simulink model "speedgoat_test_SN5659_R2021b_IO612"  (R2021b)
settings: Solver=FixedStepDiscrete  StartTime=0.0  StopTime=20  RelTol=1e-3
PreLoadFcn:
  | Ts_IO107 = 0.001;
  | Ts_IO107 = 0.001;
  | Ts_IO133 = 0.001
  | 
  | Ts_IO204 = 0.001;
  | 
  | 
  | Ts_IO503 = 0.01;
  | 
  | ts_IO612 = 1e-3;
  | Ts_IO682 = 0.005;
  | Ts_IO941 = 0.01;
InitFcn:
  | Ts_IO107 = 0.001;
  | Ts_IO107 = 0.001;
  | Ts_IO133 = 0.001
  | 
  | Ts_IO204 = 0.001;
  | 
  | 
  | Ts_IO503 = 0.01;
  | 
  | ts_IO612 = 1e-3;
  | Ts_IO682 = 0.005;
  | Ts_IO941 = 0.01;
StopFcn:
  | if isfile(['sdi_view_',bdroot,'.mldatx'])
  |  Simulink.sdi.clearPreferences();
  |  Simulink.sdi.view();
  |  pause(3);
  |  Simulink.sdi.loadView(['sdi_view_',bdroot,]);
  | end
undefined symbols (not defined in the file): C
libraries: canmsglib x12, speedgoatlib_IO612 x9, simulink x1
settings Model: Creator=yannick.orgas  LastModifiedBy=ACH
settings SolverCC: ConcurrentTasks=on  AlgebraicLoopSolver=TrustRegion  PositivePriorityOrder=on
settings DataIOCC: LimitDataPoints=on  SaveFormat=StructureWithTime
settings OptimizationCC: BlockReduction=off  OptimizeBlockIOStorage=off
settings DebuggingCC: TasksWithSamePriorityMsg=none  UnconnectedInputMsg=none  UnconnectedOutputMsg=none  UnconnectedLineMsg=none  SFMachineParentedDataDiag=warning
settings HardwareCC: ProdBitPerLong=64  ProdLongLongMode=on  ProdHWDeviceType=Intel->x86-64 (Linux 64)
settings RTWCC: Description=Simulink Real-Time  SystemTargetFile=slrealtime.tlc  TemplateMakefile=slrealtime_default_tmf  Toolchain=Simulink Real-Time Toolchain  BuildConfiguration=Faster Runs  CodeExecutionProfiling=on  TargetLang=C++
settings SimulinkRealTimeTargetCC: UseGCCFastMath=on

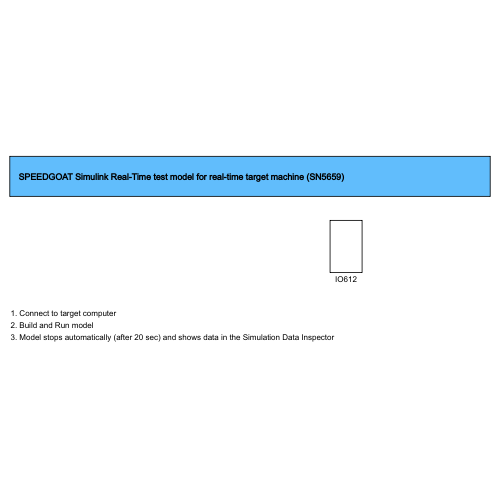
[thumbnail: Simulink's stored preview of the top-level diagram]
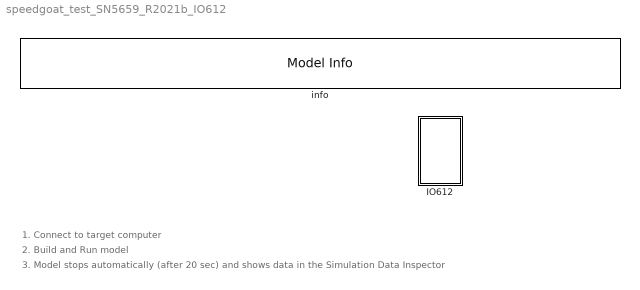
== system speedgoat_test_SN5659_R2021b_IO612 ==
  note: 1. Connect to target computer
  note: 2. Build and Run model
  note: 3. Model stops automatically (after 20 sec) and shows data in the Simulation Data Inspector
  IO612 : Subsystem
  info : simulink/Model-Wide Utilities/Model Info  Frame=on  DisplayStringWithTags=SPEEDGOAT Simulink Real-Time test model for real-time target machine (SN5659)  HorizontalTextAlignment=Left  LeftAlignmentValue=0.02

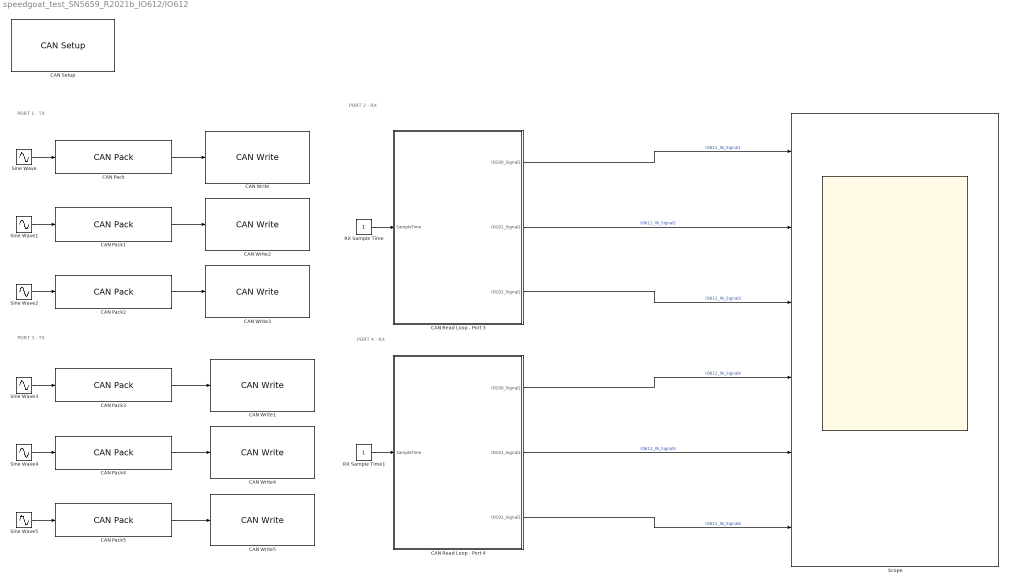
== system speedgoat_test_SN5659_R2021b_IO612/IO612 ==
  note: PORT 4 - RX
  note: PORT 1 - TX
  note: PORT 3 - TX
  note: PORT 2 - RX
  CAN Pack : canmsglib/CAN Pack  MsgList=(none)  MsgName=CAN Msg  MsgIDType=Standard (11-bit identifier)  MsgIdentifier=100  MsgLength=8  Remote=off  ApplyMinMax=off  BusOutput=off  SignalInfo={'Signal1','0','64','LE','double','Standard','0','1','0','-Inf','Inf'}
      settings: SourceProductBaseCode=ME,XP,VN  DataFormat=manually specified signals
  CAN Pack1 : canmsglib/CAN Pack  MsgList=(none)  MsgName=CAN Msg  MsgIDType=Standard (11-bit identifier)  MsgIdentifier=101  MsgLength=8  Remote=off  ApplyMinMax=off  BusOutput=off  SignalInfo={'Signal1','0','64','LE','double','Standard','0','1','0','-Inf','Inf'}
      settings: SourceProductBaseCode=ME,XP,VN  DataFormat=manually specified signals
  CAN Pack2 : canmsglib/CAN Pack  MsgList=(none)  MsgName=CAN Msg  MsgIDType=Standard (11-bit identifier)  MsgIdentifier=102  MsgLength=8  Remote=off  ApplyMinMax=off  BusOutput=off  SignalInfo={'Signal1','0','64','LE','double','Standard','0','1','0','-Inf','Inf'}
      settings: SourceProductBaseCode=ME,XP,VN  DataFormat=manually specified signals
  CAN Pack3 : canmsglib/CAN Pack  MsgList=(none)  MsgName=CAN Msg  MsgIDType=Standard (11-bit identifier)  MsgIdentifier=300  MsgLength=8  Remote=off  ApplyMinMax=off  BusOutput=off  SignalInfo={'Signal1','0','64','LE','double','Standard','0','1','0','-Inf','Inf'}
      settings: SourceProductBaseCode=ME,XP,VN  DataFormat=manually specified signals
  CAN Pack4 : canmsglib/CAN Pack  MsgList=(none)  MsgName=CAN Msg  MsgIDType=Standard (11-bit identifier)  MsgIdentifier=301  MsgLength=8  Remote=off  ApplyMinMax=off  BusOutput=off  SignalInfo={'Signal1','0','64','LE','double','Standard','0','1','0','-Inf','Inf'}
      settings: SourceProductBaseCode=ME,XP,VN  DataFormat=manually specified signals
  CAN Pack5 : canmsglib/CAN Pack  MsgList=(none)  MsgName=CAN Msg  MsgIDType=Standard (11-bit identifier)  MsgIdentifier=302  MsgLength=8  Remote=off  ApplyMinMax=off  BusOutput=off  SignalInfo={'Signal1','0','64','LE','double','Standard','0','1','0','-Inf','Inf'}
      settings: SourceProductBaseCode=ME,XP,VN  DataFormat=manually specified signals
  CAN Read Loop - Port 3 : Subsystem  TreatAsAtomicUnit=on
  CAN Read Loop - Port 4 : Subsystem  TreatAsAtomicUnit=on
  CAN Setup : speedgoatlib_IO612/CAN Setup  id=1  drvLtr=C:  PCISlot=-1  port1=CAN (HS)  port2=CAN (HS)  port3=CAN (HS)  port4=CAN (HS)  opModeCAN1=Highspeed (HS)  bdrCAN1=1 MBaud  usrBdrCAN1=[5, 1, 13, 2]  stdAccMaskCAN1=[0, 0]  extAccMaskCAN1=[0, 0]  opModeCAN2=Highspeed (HS)  bdrCAN2=1 MBaud  usrBdrCAN2=[5, 1, 13, 2]  stdAccMaskCAN2=[0, 0]  extAccMaskCAN2=[0, 0]  opModeCAN3=Highspeed (HS)  bdrCAN3=1 MBaud  usrBdrCAN3=[5, 1, 13, 2]  stdAccMaskCAN3=[0, 0]  extAccMaskCAN3=[0, 0]  opModeCAN4=Highspeed (HS)  bdrCAN4=1 MBaud  usrBdrCAN4=[5, 1, 13, 2]  stdAccMaskCAN4=[0, 0]  extAccMaskCAN4=[0, 0]  initStruct=[]  termStruct=[]  protl=IO612  qtyMod=1  chNo=[1, 2, 3, 4]  ptTypes=[1, 1, 1, 1]  protlHelpIdx=[0, 1, 2, 3]  isFDMod=0
      settings: SourceProductName=Simulink Real-Time: Speedgoat Library
  CAN Write : speedgoatlib_IO612/CAN Write  id=1  sampleTime=ts_IO612  portSelection=1  messageType=CAN  BusInput=off  enaStatusPort=off  protl=IO612  ptIdx=0  isFDMod=0
      settings: SourceProductName=Simulink Real-Time: Speedgoat Library
  CAN Write1 : speedgoatlib_IO612/CAN Write  id=1  sampleTime=ts_IO612  portSelection=3  messageType=CAN  BusInput=off  enaStatusPort=off  protl=IO612  ptIdx=2  isFDMod=0
      settings: SourceProductName=Simulink Real-Time: Speedgoat Library
  CAN Write2 : speedgoatlib_IO612/CAN Write  id=1  sampleTime=ts_IO612  portSelection=1  messageType=CAN  BusInput=off  enaStatusPort=off  protl=IO612  ptIdx=0  isFDMod=0
      settings: SourceProductName=Simulink Real-Time: Speedgoat Library
  CAN Write3 : speedgoatlib_IO612/CAN Write  id=1  sampleTime=ts_IO612  portSelection=1  messageType=CAN  BusInput=off  enaStatusPort=off  protl=IO612  ptIdx=0  isFDMod=0
      settings: SourceProductName=Simulink Real-Time: Speedgoat Library
  CAN Write4 : speedgoatlib_IO612/CAN Write  id=1  sampleTime=ts_IO612  portSelection=3  messageType=CAN  BusInput=off  enaStatusPort=off  protl=IO612  ptIdx=2  isFDMod=0
      settings: SourceProductName=Simulink Real-Time: Speedgoat Library
  CAN Write5 : speedgoatlib_IO612/CAN Write  id=1  sampleTime=ts_IO612  portSelection=3  messageType=CAN  BusInput=off  enaStatusPort=off  protl=IO612  ptIdx=2  isFDMod=0
      settings: SourceProductName=Simulink Real-Time: Speedgoat Library
  RX Sample Time : Constant  SampleTime=ts_IO612
  RX Sample Time1 : Constant  SampleTime=ts_IO612
  "Scope  " : Scope  NumInputPorts=6
  Sine Wave : Sin  Amplitude=10  Frequency=2*pi*10  SampleTime=ts_IO612
  Sine Wave1 : Sin  Amplitude=20  Frequency=2*pi*10  SampleTime=ts_IO612
  Sine Wave2 : Sin  Amplitude=30  Frequency=2*pi*10  SampleTime=ts_IO612
  Sine Wave3 : Sin  Amplitude=40  Frequency=2*pi*10  SampleTime=ts_IO612
  Sine Wave4 : Sin  Amplitude=50  Frequency=2*pi*10  SampleTime=ts_IO612
  Sine Wave5 : Sin  Amplitude=60  Frequency=2*pi*10  SampleTime=ts_IO612
  wires:
  RX Sample Time1/1 -> CAN Read Loop - Port 4/1(SampleTime)
  CAN Pack4/1 -> CAN Write4/1
  RX Sample Time/1 -> CAN Read Loop - Port 3/1(SampleTime)
  CAN Pack3/1 -> CAN Write1/1
  Sine Wave1/1 -> CAN Pack1/1
  Sine Wave4/1 -> CAN Pack4/1
  Sine Wave3/1 -> CAN Pack3/1
  Sine Wave5/1 -> CAN Pack5/1
  Sine Wave/1 -> CAN Pack/1
  Sine Wave2/1 -> CAN Pack2/1
  CAN Pack5/1 -> CAN Write5/1
  CAN Pack/1 -> CAN Write/1
  CAN Pack1/1 -> CAN Write2/1
  CAN Pack2/1 -> CAN Write3/1
  CAN Read Loop - Port 3/1(ID100_Signal1) -> "Scope  "/1  "IO612_IN_Signal1"
  CAN Read Loop - Port 3/2(ID101_Signal1) -> "Scope  "/2  "IO612_IN_Signal2"
  CAN Read Loop - Port 3/3(ID102_Signal1) -> "Scope  "/3  "IO612_IN_Signal3"
  CAN Read Loop - Port 4/1(ID100_Signal1) -> "Scope  "/4  "IO612_IN_Signal4"
  CAN Read Loop - Port 4/2(ID101_Signal1) -> "Scope  "/5  "IO612_IN_Signal5"
  CAN Read Loop - Port 4/3(ID102_Signal1) -> "Scope  "/6  "IO612_IN_Signal6"

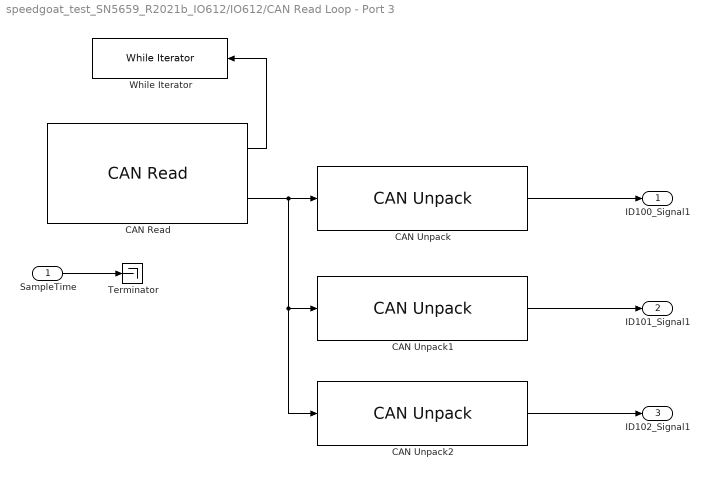
== system speedgoat_test_SN5659_R2021b_IO612/IO612/CAN Read Loop - Port 3 ==
  SampleTime : Inport
  CAN Read : speedgoatlib_IO612/CAN Read  id=1  sampleTime=-1  portSelection=2  messageType=CAN  BusOutput=off  protl=IO612  ptIdx=1  isFDMod=0
      settings: SourceProductName=Simulink Real-Time: Speedgoat Library
  CAN Unpack : canmsglib/CAN Unpack  MsgList=(none)  MsgName=CAN Msg  MsgIDType=Standard (11-bit identifier)  MsgIdentifier=100  MsgLength=8  SignalInfo={'Signal1','0','64','LE','double','Standard','0','1','0','-Inf','Inf'}  IDPort=off  TimestampPort=off  ErrorPort=off  RemotePort=off  LengthPort=off  StatusPort=off  ApplyMinMax=off
      settings: SourceProductBaseCode=ME,XP,VN
  CAN Unpack1 : canmsglib/CAN Unpack  MsgList=(none)  MsgName=CAN Msg  MsgIDType=Standard (11-bit identifier)  MsgIdentifier=101  MsgLength=8  SignalInfo={'Signal1','0','64','LE','double','Standard','0','1','0','-Inf','Inf'}  IDPort=off  TimestampPort=off  ErrorPort=off  RemotePort=off  LengthPort=off  StatusPort=off  ApplyMinMax=off
      settings: SourceProductBaseCode=ME,XP,VN
  CAN Unpack2 : canmsglib/CAN Unpack  MsgList=(none)  MsgName=CAN Msg  MsgIDType=Standard (11-bit identifier)  MsgIdentifier=102  MsgLength=8  SignalInfo={'Signal1','0','64','LE','double','Standard','0','1','0','-Inf','Inf'}  IDPort=off  TimestampPort=off  ErrorPort=off  RemotePort=off  LengthPort=off  StatusPort=off  ApplyMinMax=off
      settings: SourceProductBaseCode=ME,XP,VN
  Terminator : Terminator
  While Iterator : WhileIterator  MaxIters=501  WhileBlockType=do-while
  ID100_Signal1 : Outport
  ID101_Signal1 : Outport  Port=2
  ID102_Signal1 : Outport  Port=3
  wires:
  SampleTime/1 -> Terminator/1
  CAN Unpack2/1 -> ID102_Signal1/1
  CAN Unpack1/1 -> ID101_Signal1/1
  CAN Unpack/1 -> ID100_Signal1/1
  CAN Read/1 -> While Iterator/1
  CAN Read/2 -> CAN Unpack/1, CAN Unpack1/1, CAN Unpack2/1

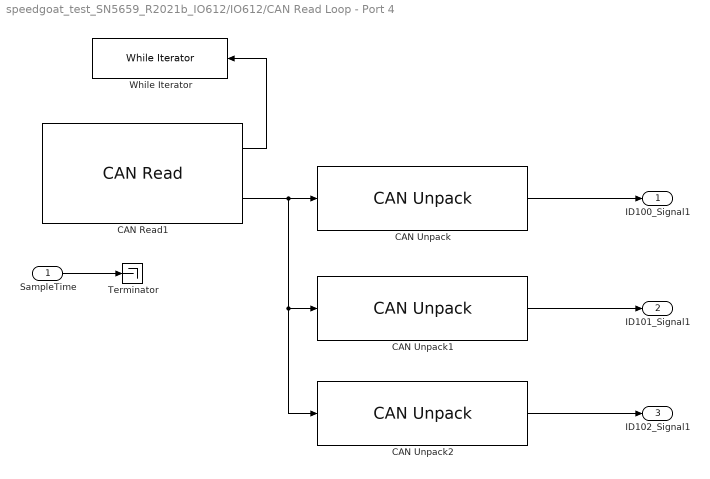
== system speedgoat_test_SN5659_R2021b_IO612/IO612/CAN Read Loop - Port 4 ==
  SampleTime : Inport
  CAN Read1 : speedgoatlib_IO612/CAN Read  id=1  sampleTime=-1  portSelection=4  messageType=CAN  BusOutput=off  protl=IO612  ptIdx=3  isFDMod=0
      settings: SourceProductName=Simulink Real-Time: Speedgoat Library
  CAN Unpack : canmsglib/CAN Unpack  MsgList=(none)  MsgName=CAN Msg  MsgIDType=Standard (11-bit identifier)  MsgIdentifier=300  MsgLength=8  SignalInfo={'Signal1','0','64','LE','double','Standard','0','1','0','-Inf','Inf'}  IDPort=off  TimestampPort=off  ErrorPort=off  RemotePort=off  LengthPort=off  StatusPort=off  ApplyMinMax=off
      settings: SourceProductBaseCode=ME,XP,VN
  CAN Unpack1 : canmsglib/CAN Unpack  MsgList=(none)  MsgName=CAN Msg  MsgIDType=Standard (11-bit identifier)  MsgIdentifier=301  MsgLength=8  SignalInfo={'Signal1','0','64','LE','double','Standard','0','1','0','-Inf','Inf'}  IDPort=off  TimestampPort=off  ErrorPort=off  RemotePort=off  LengthPort=off  StatusPort=off  ApplyMinMax=off
      settings: SourceProductBaseCode=ME,XP,VN
  CAN Unpack2 : canmsglib/CAN Unpack  MsgList=(none)  MsgName=CAN Msg  MsgIDType=Standard (11-bit identifier)  MsgIdentifier=302  MsgLength=8  SignalInfo={'Signal1','0','64','LE','double','Standard','0','1','0','-Inf','Inf'}  IDPort=off  TimestampPort=off  ErrorPort=off  RemotePort=off  LengthPort=off  StatusPort=off  ApplyMinMax=off
      settings: SourceProductBaseCode=ME,XP,VN
  Terminator : Terminator
  While Iterator : WhileIterator  MaxIters=501  WhileBlockType=do-while
  ID100_Signal1 : Outport
  ID101_Signal1 : Outport  Port=2
  ID102_Signal1 : Outport  Port=3
  wires:
  CAN Read1/2 -> CAN Unpack2/1, CAN Unpack1/1, CAN Unpack/1
  CAN Read1/1 -> While Iterator/1
  CAN Unpack/1 -> ID100_Signal1/1
  CAN Unpack1/1 -> ID101_Signal1/1
  CAN Unpack2/1 -> ID102_Signal1/1
  SampleTime/1 -> Terminator/1
